simulink library "mpc555drivers"  (Simulink 6.0)
settings: Solver=ode45  SolverMode=SingleTasking  StartTime=0.0  StopTime=10.0  RelTol=1e-3
PreLoadFcn:
  | RTWConfigurationCB('preloadfcn', bdroot);
InitFcn:
  | % START RTW CONFIGURATION CODE %
  | RTWConfigurationCB('rtw_target_initfcn',gcs);
  | % END RTW CONFIGURATION CODE %
undefined symbols (not defined in the file or in its folder): pmax, scale
libraries: passthrough x52, driver_interface_library x18, mpc555toucan x11, mpc555extras x9, config_library x7, exprofilelib x4, simulink x3, mpc555drivers x2, canblocks x1
(part 1 of 3)
settings Model: Creator=The MathWorks Inc.  LastModifiedBy=batserve  ExtModeAutoUpdateStatusClock=off  ProdHWDeviceType=Specified
settings DataIOCC: SignalLoggingName=logsOut
settings OptimizationCC: BooleanDataType=off
settings DebuggingCC: CheckExecutionContextPreStartOutputMsg=on  CheckExecutionContextRuntimeOutputMsg=on  SolverPrmCheckMsg=none
settings HardwareCC: ProdHWDeviceType=Specified  TargetUnknown=on
settings ModelReferenceCC: UpdateModelReferenceTargets=IfOutOfDate

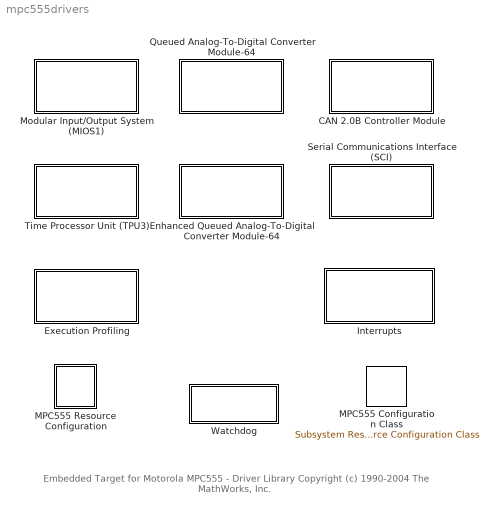
== system mpc555drivers ==
  note: Embedded Target for Motorola MPC555 - Driver Library
      | Copyright (c) 1990-2004 The MathWorks, Inc.
  CAN 2.0B Controller Module : Subsystem  PropExecContextAcrossSSBoundary=on
      mask Display: disp('TouCAN')
  Enhanced Queued Analog-To-Digital Converter Module-64 : Subsystem  PropExecContextAcrossSSBoundary=on
      mask Display: disp('QADC64E\n(MPC565/566)')
  Execution Profiling : Subsystem  PropExecContextAcrossSSBoundary=on
      mask Display: disp('Execution\nProfiling')
  Interrupts : Subsystem  PropExecContextAcrossSSBoundary=on
      settings: OpenFcn=mpc555interrupts
      mask Display: disp('Interrupt Handling')
  MPC555 Configuration Class : config_library/Subsystem Resource Configuration Class  Tag=CONFIGURATION DATA CLASS  dClassName=MPC555dkConfig.SYSTEM_CLOCKS  rClassName=MPC555dkConfig.SystemResources
  MPC555 Resource Configuration : Subsystem  Tag=RTW CONFIGURATION BLOCK  AncestorBlock=|  PropExecContextAcrossSSBoundary=on  mask(Subsystem Resource Configuration){oldParentName=, oldBlockName=, defaultConfigLibrary=}
      | config_library/Subsystem
      | Resource
      | Configuration
      mask prompts: oldParentName "Old Parent Name"; oldBlockName "Old Block Name"; defaultConfigLibrary "Default Configuration Library"
      settings: CopyFcn=RTWConfigurationCB('copyfcn',gcb);  DeleteFcn=RTWConfigurationCB('deletefcn',gcb);  UndoDeleteFcn=RTWConfigurationCB('NameChangeFcn',gcb);  PreSaveFcn=RTWConfigurationCB('presavefcn',gcb);  NameChangeFcn=RTWConfigurationCB('NameChangeFcn',gcb);  OpenFcn=RTWConfigurationCB('openfcn',gcb);
      mask Display: image(imread('target_icon.jpg'))
  Modular Input/Output System (MIOS1) : Subsystem  PropExecContextAcrossSSBoundary=on
      mask Display: disp(sprintf('MIOS1 / MIOS14'))
  Queued Analog-To-Digital Converter Module-64 : Subsystem  PropExecContextAcrossSSBoundary=on
      mask Display: disp('QADC64\n(MPC555)')
  Serial Communications Interface (SCI) : Subsystem  PropExecContextAcrossSSBoundary=on
      mask Display: disp('Serial')
  Time Processor Unit (TPU3) : Subsystem  PropExecContextAcrossSSBoundary=on
      mask Display: disp('TPU3')
  Watchdog : Subsystem  PropExecContextAcrossSSBoundary=on  mask(MPC555 Watchdog){timeout=0.1}
      mask prompts: timeout "Watchdog Timeout [seconds]"
      mask help:
      | Set the timeout period of the watchdog timer.
      |
      | Normally the timer is reset every time the fastest sample period of the model executes. If the model gets locked and stops executing then the watchdog will timeout and reset the processor.
      mask init:
      | [model_init_function_code] = mask_mpc555_watchdog('initfcn',gcb,timeout);
      mask Help: helpview([docroot '/toolbox/mpc555dk/mpc555dk.map'], 'Bow_Wow');
      mask CallbackString:
      | timeout = eval(get_param(gcb,'timeout'),[]);
      | % If eval returns empty, then it may be that a variable was
      | % specified rather than a numeric value. We can only do the range
      | % check at this point if a numeric value was entered.
      | if ~isempty(timeout)
      | 	timeout = mask_mpc555_watchdog('rangecheck',gcb,timeout);
      | end
      mask Display: disp('Watchdog \nTimer')

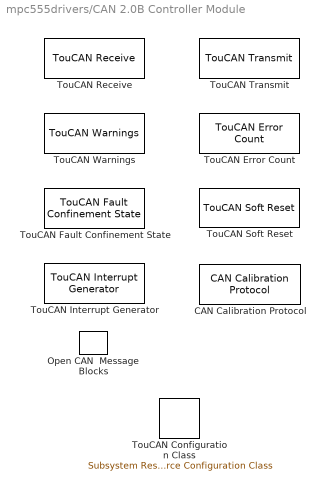
== system mpc555drivers/CAN 2.0B Controller Module ==
  CAN Calibration Protocol : mpc555toucan/CAN Calibration Protocol  CCP_STATION_ID=hex2dec('1')  module=A  ccp_cro_id=hex2dec('6FA')  ccp_cro_message_type=Extended (29-bit identifier)  ccp_return_id=hex2dec('6FB')  ccp_return_message_type=Extended (29-bit identifier)  TOTAL_NUM_ODTS=8  cro_sample_time=0.01
  Open CAN  Message Blocks : mpc555toucan/Open CAN  Message Blocks
  TouCAN Configuration Class : config_library/Subsystem Resource Configuration Class  Tag=CONFIGURATION DATA CLASS  dClassName=MPC555dkConfig.TOUCAN  rClassName=MPC555dkConfig.TOUCAN_RESOURCES
  TouCAN Error Count : mpc555toucan/TouCAN Error Count  module=A  t=0.1  enablePassThru=off
  TouCAN Fault Confinement State : mpc555toucan/TouCAN Fault Confinement State  module=A  t=0.1  enablePassThru=off
  TouCAN Interrupt Generator : mpc555toucan/TouCAN Interrupt Generator  module=A  callback=Error  float_flag=on
  TouCAN Receive : mpc555toucan/TouCAN Receive  module=A  ids=hex2dec('0001')  notification_type=Function Call Outport  auto_select_buffer=on  bufferids=14  use_queue=off  queue_length=3  message_type=Standard (11-bit identifier)  t=0.1
  TouCAN Soft Reset : mpc555toucan/TouCAN Soft Reset  module=A  t=-1
  TouCAN Transmit : mpc555toucan/TouCAN Transmit  module=A  tx_mode=Queued transmission with shared buffer  fifo_queue_length=8  bufferids=0  t=-1  enablePassThru=off
  TouCAN Warnings : mpc555toucan/TouCAN Warnings  module=A  t=0.1  enablePassThru=off

== system mpc555drivers/Enhanced Queued Analog-To-Digital Converter Module-64 ==
  QADCE Configuration Class : config_library/Subsystem Resource Configuration Class  Tag=CONFIGURATION DATA CLASS  dClassName=MPC555dkConfig.QADC64E  rClassName=MPC555dkConfig.QADC_Resources
  QADCE Analog In : Subsystem  PropExecContextAcrossSSBoundary=on  mask(MPC555 Analog Input (Enhanced QADC64, Continuous-scan)){module=A, channels=[ 44 45 46 47 64 65 66 ], justification=Right-justified (unsigned), t=0.1}
      mask prompts: module "QADCE module:"; t "Sample time:"
      mask help:
      | Analog input using one of the Queued Analog Digital Converter (QADC64) modules. The module is operated in continuous-scan mode.
      |
      | Specifying channel numbers:
      | - In non-multiplexed mode, specify the channels as a vector of numbers from [44..59, 64..87], correponding to pins AN44..AN59 and AN64..AN87.
      | - In multiplexed mode see the table in the documentation.
      mask init:
      | % check for a Resource Config block, and make sure it is MPC555
      | target = RTWConfigurationCB('get_target', gcb);
      | target.checkName('MPC555');
      | 
      | num_channels = length(channels);
      | register = mask_qadce_analogue_in(module,channels,justification);
      | 
      | if justification == 3
      |     outDType = 'int16';
      | else
      |    outDType = 'uint16';
      | end
      | 
      | % check for a valid target block
      | driverBlock = regexprep(gcb, sprintf('\n'), ' ');
      | target = RTWConfigurationCB('get_target', driverBlock);
      | 
      | % Perform Resource Configuration
      | RTWConfiguration.Target.acquireResourceForBlock(      ...
      |    gcb,                    ...   % Current block
      |    'MPC555dkConfig.QADC64E', ...   % Configuration Class
      |    'QADC_MODULES',          ...   % Resource Type associated with the configuration class
      |    module,                    ...   % Resource being requested
      |    'QADC Module'            ...   % Lable to be used in error messages
      | );
      mask Help: helpview([docroot '/toolbox/mpc555dk/mpc555dk.map'], 'QADCE_An_In');
      mask StyleString: popup(A|B),edit,popup(Right-justified (unsigned)|Left-justified (unsigned)|Left-justified (signed)),edit
      mask Display: disp(sprintf('Analog In\n(QADCE_%s)',module));
  QADCE Digital In : Subsystem  PropExecContextAcrossSSBoundary=on  mask(MPC555 Digital Input (Enhanced QADC64)){module=A, port=A, bits=[0 1 2 3], t=0.1}
      mask prompts: module "QADC module:"; t "Sample time:"
      mask help:
      | Digital input using one of the Queued Analog Digital Converter (QADC64) modules.
      |
      | Specify the bits you want to read as a vector of numbers from [0..7]. Depending on the selected port, the bits entered correspond to pins:
      | - PQA0..PQA7 (Port A)
      | - PQB0..PQB7 (Port B)
      mask init:
      | % check for a Resource Config block, and make sure it is MPC555
      | target = RTWConfigurationCB('get_target', gcb);
      | target.checkName('MPC555');
      | 
      | % check for a valid target block
      | driverBlock = regexprep(gcb, sprintf('\n'), ' ');
      | target = RTWConfigurationCB('get_target', driverBlock);
      | 
      | %parameter check
      | permitted = 0:7;
      | if any( ~ismember(bits,permitted) )
      |   error(['At least one illegal bit number number was specified. The permitted bit numbers are '...
      |          num2str(permitted) '. Check that all specified bit numbers are in this set.']);
      | end
      | 
      | % The Digital In Register To Read
      | register=['QADC_' module '.PORTQ' port '.R'];
      | 
      | % The Masks
      | masks = bitshift(1,bits,8);
      | 
      | % Perform Resource Configuration
      | for i = 1:length(bits)
      | 	pins{i} = sprintf('%d', bits(i));
      | end
      | resource = ['QADC_' module '_DIGITAL_PORT' port ];
      | RTWConfiguration.Target.acquireResourceForBlock(      ...
      |    gcb,                    ...   % Current block
      |    'MPC555dkConfig.QADC64E', ...   % Configuration Class
      |    resource,          ...   % Resource Type associated with the configuration class
      |    pins,                    ...   % Resources being requested
      |    'QADC Digital Input Pin(s)'            ...   % Lable to be used in error messages
      | );
      mask Help: helpview([docroot '/toolbox/mpc555dk/mpc555dk.map'], 'QADCE_Dig_In');
      mask StyleString: popup(A|B),popup(A|B),edit,edit
      mask Display: disp(sprintf('Digital In\n(QADCE_%s)',module));

== system mpc555drivers/Execution Profiling ==
  MPC555 Execution Profiling via CAN A : Subsystem  TreatAsAtomicUnit=on  PropExecContextAcrossSSBoundary=on  mask(MPC555 Execution Profiling via CAN Channel A){commandId=hex2dec('1FFFFF00'), execCopyFcn=on, dataId=hex2dec('1FFFFF01'), t=1}
      mask prompts: commandId "Start command CAN message identifier:"; execCopyFcn "Execute CopyFcn"; dataId "Returned data CAN message identifier:"; t "Sample time:"
      mask help:
      | Provides a CAN interface to the execution profiling engine. On receipt of a start command message, logging of execution profile data begins. On completion of a logging run, the recorded data is automatically returned via CAN.
      |
      | You must specify the message identifiers for the start command and the returned data. These identifiers must be compatible with the values used by the host-side part of the execution profiling utility. See also the MATLAB command profile_mpc555.
      mask init:
      | % check for a Resource Config block, and make sure it is MPC555
      | target = RTWConfigurationCB('get_target', gcb);
      | target.checkName('MPC555');
      settings: CopyFcn=exprofile_copyfcn(gcb);
      mask Help: helpview([docroot '/toolbox/mpc555dk/mpc555dk.map'], 'Execution_Profiling_Can_A');
      mask Display: disp('Execution Profiling\nvia CAN')
  MPC555 Execution Profiling via SCI1 : Subsystem  TreatAsAtomicUnit=on  PropExecContextAcrossSSBoundary=on  mask(MPC555  Execution Profiling via Serial Port SCI1){t=1, execCopyFcn=on}
      mask prompts: t "Sample time:"; execCopyFcn "Execute CopyFcn"
      mask help:
      | Provides a serial interface to the execution profiling engine. On receipt of a start command to the serial port, logging of execution profile data begins. On completion of a logging run, the recorded data is automatically returned via serial.
      |
      | No other serial blocks may be used in the model if an MPC555 Execution Profiling via SCI1 block is present.
      |
      | See also the MATLAB command profile_mpc555.
      mask init:
      | % check for a Resource Config block, and make sure it is MPC555
      | target = RTWConfigurationCB('get_target', gcb);
      | target.checkName('MPC555');
      settings: CopyFcn=exprofile_copyfcn(gcb);
      mask Help: helpview([docroot '/toolbox/mpc555/mpc555.map'], 'Execution_Profiling_SCI1');
      mask Display: disp('Execution Profiling\nvia Serial')

== system mpc555drivers/Interrupts ==

== system mpc555drivers/MPC555 Resource Configuration ==
  config : S-Function  FunctionName=sfunRTWConfig

== system mpc555drivers/Modular Input/Output System (MIOS1) ==
  MIOS Configuration Class : config_library/Subsystem Resource Configuration Class  Tag=CONFIGURATION DATA CLASS  dClassName=MPC555dkConfig.MIOS1  rClassName=MPC555dkConfig.MiosResources
  MIOS Digital In : Subsystem  PropExecContextAcrossSSBoundary=on  mask(MPC555 Digital Input (MPIOSM)){bits=[0 1 2], t=0.1, enablePassThru=off}
      mask prompts: t "Sample time:"; enablePassThru "Enable pass through (show simulation input)"
      mask help:
      | Reads the logical state of specified pins on the MIOS 16-bit parallel port I/O submodule (MPIOSM).
      |
      | Specify the bits you want to read as a vector of numbers from [0..15], corresponding to pins MPIO32B0..MPIO32B15.
      mask init:
      | simulinkPortControl(gcbh,'enable','PassThrough',enablePassThru);
      | 
      | %Deprecation warning for passthrough
      | if (enablePassThru)
      | 	passThroughDeprecationWarning;
      | end;
      | 
      | % check for a Resource Config block, and make sure it is MPC555
      | target = RTWConfigurationCB('get_target', gcb);
      | target.checkName('MPC555');
      | 
      | mpc555_mask_mios_dig_io('init', gcb, bits);
      | masks=uint16(bitshift(1,bits));
      | bits=int16(bits); % Prevent decimal points in generated code.
      mask Help: helpview([docroot '/toolbox/mpc555dk/mpc555dk.map'], 'MIOS_Dig_In');
      mask CallbackString: mpc555_mask_mios_dig_io('callback', gcb);||
      mask Display: disp(['Digital In\n(MPIOSM)'])
  MIOS Digital Out : Subsystem  PropExecContextAcrossSSBoundary=on  mask(MPC555 Digital Output (MPIOSM)){bits=[0 1], init=0, t=-1, enablePassThru=off}
      mask prompts: init "Initial output level:"; t "Sample time:"; enablePassThru "Enable pass through (show simulation output)"
      mask help:
      | Sets the logical state of specified pins on the MIOS 16-bit parallel port I/O submodule (MPIOSM). When the input signal is greater than zero a logical one is written to the corresponding pin; otherwise a logical zero is written.
      |
      | Specify the bits you want to set as a vector of numbers from [0..15], corresponding to pins MPIO32B0..MPIO32B15.
      mask init:
      | simulinkPortControl(gcbh,'enable','PassThrough',enablePassThru);
      | 
      | %Deprecation warning for passthrough
      | if (enablePassThru)
      | 	passThroughDeprecationWarning;
      | end;
      | 
      | bits = double(bits);
      | init = double(init~=0);
      | 
      | % Check the init and bits parameters for the correct length
      | if length(init) == 1
      | 	init = repmat(init,1,length(bits));
      | elseif length(init) ~= length(bits)
      | 	error('''Initial Output Level'' parameter must either be a scalar or the same length as the ''bits'' parameter.');
      | end
      | 
      | % check for a Resource Config block, and make sure it is MPC555
      | target = RTWConfigurationCB('get_target', gcb);
      | target.checkName('MPC555');
      | 
      | mpc555_mask_mios_dig_io('init', gcb, bits);
      | masks=uint16(bitshift(1,bits));
      mask Help: helpview([docroot '/toolbox/mpc555dk/mpc555dk.map'], 'MIOS_Dig_Out');
      mask CallbackString: mpc555_mask_mios_dig_io('callback', gcb);|||
      mask Display: disp(['Digital Out\n (MPIOSM)'])
  MIOS Digital Out (MPWMSM) : Subsystem  Priority=2  PropExecContextAcrossSSBoundary=on  mask(MPC555 Digital Output (MPWMSM)){module=0, init=0, t=-1, enablePassThru=off}
      mask prompts: module "MPWM submodule number:"; init "Initial output level:"; t "Sample time:"; enablePassThru "Enable pass through (show simulation output)"
      mask help:
      | Configures a MIOS pulse width modulation submodule (MPWMSM) for use as digital output. When the input signal is greater than zero a logical one is written to the output pin; otherwise a logical zero is written.
      |
      | This block outputs on one of the pins MPWM0..MPWM3 or MPWM16..MPWM19.
      mask init:
      | simulinkPortControl(gcbh,'enable','PassThrough',enablePassThru);
      | 
      | %Deprecation warning for passthrough
      | if (enablePassThru)
      | 	passThroughDeprecationWarning;
      | end;
      | 
      | % check for a Resource Config block, and make sure it is MPC555
      | target = RTWConfigurationCB('get_target', gcb);
      | target.checkName('MPC555');
      | 
      | init = init ~= 0;
      | 
      | % MIOS14 has 4 more PWM channels than the MIOS1
      | if ismember(module, {'4' '5' '20' '21'} ) && ...
      |    ~mpc555_module_available(mpc5xx_get_target_variant(gcb),'MIOS14')
      | 	msg = sprintf('\n\nPWM module %s is not available.\nModules { 4 5 20 21 } are only supported on processor variants with a MIOS14 module.\nPlease choose a different module or a different processor variant',module);
      | 	error(msg);
      | end
      | 
      | % Perform Resource Configuration
      | RTWConfiguration.Target.acquireResourceForBlock(      ...
      |    gcb,                    ...   % Current block
      |    'MPC555dkConfig.MIOS1', ...   % Configuration Class
      |    'PWM_MODULES',          ...   % Resource Type associated with the configuration class
      |    module,                    ...   % Resource being requested
      |    'PWM Module'            ...   % Label to be used in error messages
      | );
      mask Help: helpview([docroot '/toolbox/mpc555dk/mpc555dk.map'], 'MIOS_Dig_Out_MPWMSM');
      mask StyleString: popup(0|1|2|3|4|5|16|17|18|19|20|21),popup(0|1),edit,checkbox
      mask Display: disp('Digital Out\n(MPWMSM)')
  MIOS Pulse Width Modulation Out : Subsystem  Priority=2  PropExecContextAcrossSSBoundary=on  mask(MPC555 Pulse Width Modulation Output (MPWMSM)){module=0, timing_settings=off, period=0.0375, initpw=0.5, cp=, pp=, t=-1, pol=off, trsp=off, fren=off, enablePassThru=off}
      mask prompts: module "MPWM submodule number:"; timing_settings "Edit period registers manually"; period "Ideal period (sec):"; initpw "Initial duty cycle (0 <= duty cycle <= 1):"; cp "Clock prescaler field of MPWMSM Status/Control Register:"; pp "Number of clock ticks per period:"; t "Sample time:"; pol "Invert output polarity"; trsp "Activate transparent mode"; fren "Hold output when at debug breakpoint (freeze enable)"; enablePassThru "Enable pass through (show simulation output)"
      mask help:
      | Configures a MIOS pulse width modulation submodule (MPWMSM) to generate a pulse width modulated output signal.
      |
      | This block outputs on one of the pins MPWM0..MPWM3 or MPWM16..MPWM19.
      mask init:
      | simulinkPortControl(gcbh,'enable','PassThrough',enablePassThru);
      | 
      | %Deprecation warning for passthrough
      | if (enablePassThru)
      | 	passThroughDeprecationWarning;
      | end;
      | 
      | % check for a Resource Config block, and make sure it is MPC555
      | target = RTWConfigurationCB('get_target', gcb);
      | target.checkName('MPC555');
      | 
      | % Calculate period
      | [period,cp,pp] = mask_pwm_config('period_calc',gcb,period,cp,pp);
      | 
      | % Verify Initial pulse width
      | if initpw > 1 || initpw < 0
      | 	error('Initial Pulse Width Parameter ( pw ) must satisfy 0 <= pw <= 1');
      | end
      | % Calculate the initial value for the PULR register
      | initpw = round(pp * initpw);
      | 
      | % MIOS14 has 4 more PWM channels than the MIOS1
      | if ismember(module, {'4' '5' '20' '21'} ) && ...
      |    ~mpc555_module_available(mpc5xx_get_target_variant(gcb),'MIOS14')
      | 	msg = sprintf('\n\nPWM module %s is not available.\nModules { 4 5 20 21 } are only supported on processor variants with a MIOS14 module.\nPlease choose a different module or a different processor variant',module);
      | 	error(msg);
      | end
      | 
      | % Perform Resource Configuration
      | RTWConfiguration.Target.acquireResourceForBlock(      ...
      |    gcb,                    ...   % Current block
      |    'MPC555dkConfig.MIOS1', ...   % Configuration Class
      |    'PWM_MODULES',          ...   % Resource Type associated with the configuration class
      |    module,                    ...   % Resource being requested
      |    'PWM Module'            ...   % Lable to be used in error messages
      | );
      mask Help: helpview([docroot '/toolbox/mpc555dk/mpc555dk.map'], 'MIOS_PWM');
      mask StyleString: popup(0|1|2|3|4|5|16|17|18|19|20|21),checkbox,edit,edit,edit,edit,edit,checkbox,checkbox,checkbox,checkbox
      mask CallbackString: |mask_pwm_config('timing_settings',gcb)|mask_pwm_config('period_update',gcb)||mask_pwm_config('period_update',gcb)|mask_pwm_config('period_update',gcb)|||||
      mask Display: disp('PWM Out\n(MPWMSM)')
  MIOS Waveform Measurement : Subsystem  PropExecContextAcrossSSBoundary=on  mask(MPC555 Waveform Measurement (MDASM)){module=11, operation=Pulse width, bsl=Counter Bus 6 (CB6), range=[ 1e-006 , 0.065536 ], t=0.1, edpol=off, fren=off, enablePassThru=off}
      mask prompts: module "MDASM submodule number:"; operation "Measurement:"; bsl "Counter bus:"; range "Measurement range: [ resolution, max] seconds"; t "Sample time:"; edpol "Invert input polarity"; fren "Hold internal counters when at debug breakpoint (freeze enable)"; enablePassThru "Enable pass through (show simulation input)"
      mask help:
      | Configures the MIOS double action submodule (MDASM) for pulse width or pulse period measurement.
      |
      | This block inputs on one of the pins MDA11..MDA15 or MDA27..MDA31.
      mask init:
      | simulinkPortControl(gcbh,'enable','PassThrough',enablePassThru);
      | 
      | %Deprecation warning for passthrough
      | if (enablePassThru)
      | 	passThroughDeprecationWarning;
      | end;
      | 
      | % check for a Resource Config block, and make sure it is MPC555
      | target = RTWConfigurationCB('get_target', gcb);
      | target.checkName('MPC555');
      | 
      | % scale and pmax are
      | % all used under the mask
      | [scale, pmax, pmin] = mask_mdasm_ipwm('code',gcb);
      | 
      | % Perform Resource Configuration
      | RTWConfiguration.Target.acquireResourceForBlock(      ...
      |    gcb,                    ...   % Current block
      |    'MPC555dkConfig.MIOS1', ...   % Configuration Class
      |    'MDASM_MODULES',          ...   % Resource Type associated with the configuration class
      |    module,                    ...   % Resource being requested
      |    'MDASM Module'            ...   % Lable to be used in error messages
      | );
      mask Help: helpview([docroot '/toolbox/mpc555dk/mpc555dk.map'], 'Waveform_Measurement');
      mask StyleString: popup(11|12|13|14|15|27|28|29|30|31),popup(Pulse width|Pulse period),popup(Counter Bus 6 (CB6)|Counter Bus 22 (CB22)),edit,edit,checkbox,checkbox,checkbox
      mask CallbackString: ||mask_mdasm_ipwm('update_range', gcb);|||||
      mask Display: disp('Pulse Width\n(MDASM)');

== system mpc555drivers/Queued Analog-To-Digital Converter Module-64 ==
  QADC Configuration Class : config_library/Subsystem Resource Configuration Class  Tag=CONFIGURATION DATA CLASS  dClassName=MPC555dkConfig.QADC64  rClassName=MPC555dkConfig.QADC_Resources
  QADC Analog In : Subsystem  PropExecContextAcrossSSBoundary=on  mask(MPC555 Analog Input (QADC64, Continuous-scan)){module=A, channels=[0 1 2 3 48 49 50 51], justification=Right-justified (unsigned), t=0.1, enablePassThru=off}
      mask prompts: module "QADC module:"; t "Sample time:"; enablePassThru "Enable pass through (show simulation input)"
      mask help:
      | Analog input using one of the Queued Analog Digital Converter (QADC64) modules. The module is operated in continuous-scan mode.
      |
      | Specifying channel numbers:
      | - In non-multiplexed mode, specify the channels as a vector of numbers from [0..3, 48..59], correponding to pins AN0..AN3 and AN48..AN59.
      | - In multiplexed mode see the table in the documentation.
      mask init:
      | simulinkPortControl(gcbh,'enable','PassThrough',enablePassThru);
      | 
      | %Deprecation warning for passthrough
      | if (enablePassThru)
      | 	passThroughDeprecationWarning;
      | end;
      | 
      | % check for a Resource Config block, and make sure it is MPC555
      | target = RTWConfigurationCB('get_target', gcb);
      | target.checkName('MPC555');
      | 
      | num_channels = length(channels);
      | register = mask_qadc_analogue_in(module,channels,justification);
      | 
      | if justification == 3
      |     outDType = 'int16';
      | else
      |    outDType = 'uint16';
      | end
      | 
      | % check for a valid target block
      | driverBlock = regexprep(gcb, sprintf('\n'), ' ');
      | target = RTWConfigurationCB('get_target', driverBlock);
      | 
      | % Perform Resource Configuration
      | RTWConfiguration.Target.acquireResourceForBlock(      ...
      |    gcb,                    ...   % Current block
      |    'MPC555dkConfig.QADC64', ...   % Configuration Class
      |    'QADC_MODULES',          ...   % Resource Type associated with the configuration class
      |    module,                    ...   % Resource being requested
      |    'QADC Module'            ...   % Lable to be used in error messages
      | );
      mask Help: helpview([docroot '/toolbox/mpc555dk/mpc555dk.map'], 'QADC_An_In');
      mask StyleString: popup(A|B),edit,popup(Right-justified (unsigned)|Left-justified (unsigned)|Left-justified (signed)),edit,checkbox
      mask Display: disp(sprintf('Analog In\n(QADC_%s)',module));
  QADC Digital In : Subsystem  PropExecContextAcrossSSBoundary=on  mask(MPC555 Digital Input (QADC64)){module=A, port=A, bits=[0 1 2 3], t=0.1, enablePassThru=off}
      mask prompts: module "QADC module:"; t "Sample time:"; enablePassThru "Enable pass through (show simulation input)"
      mask help:
      | Digital input using one of the Queued Analog Digital Converter (QADC64) modules.
      |
      | Specify the bits you want to read as a vector of numbers from [0..7]. Depending on the selected port, the bits entered correspond to pins:
      | - PQA0..PQA7 (Port A)
      | - PQB0..PQB7 (Port B)
      mask init:
      | simulinkPortControl(gcbh,'enable','PassThrough',enablePassThru);
      | 
      | %Deprecation warning for passthrough
      | if (enablePassThru)
      | 	passThroughDeprecationWarning;
      | end;
      | 
      | % check for a Resource Config block, and make sure it is MPC555
      | target = RTWConfigurationCB('get_target', gcb);
      | target.checkName('MPC555');
      | 
      | % check for a valid target block
      | driverBlock = regexprep(gcb, sprintf('\n'), ' ');
      | target = RTWConfigurationCB('get_target', driverBlock);
      | 
      | %parameter check
      | permitted = 0:7;
      | if any( ~ismember(bits,permitted) )
      |   error(['At least one illegal bit number number was specified. The permitted bit numbers are '...
      |          num2str(permitted) '. Check that all specified bit numbers are in this set.']);
      | end
      | 
      | % The Digital In Register To Read
      | register=['QADC_' module '.PORTQ' port '.R'];
      | 
      | % The Masks
      | masks = bitshift(1,bits,8);
      | 
      | % Perform Resource Configuration
      | for i = 1:length(bits)
      | 	pins{i} = sprintf('%d', bits(i));
      | end
      | resource = ['QADC_' module '_DIGITAL_PORT' port ];
      | RTWConfiguration.Target.acquireResourceForBlock(      ...
      |    gcb,                    ...   % Current block
      |    'MPC555dkConfig.QADC64', ...   % Configuration Class
      |    resource,          ...   % Resource Type associated with the configuration class
      |    pins,                    ...   % Resources being requested
      |    'QADC Digital Input Pin(s)'            ...   % Lable to be used in error messages
      | );
      mask Help: helpview([docroot '/toolbox/mpc555dk/mpc555dk.map'], 'QADC_Dig_In');
      mask StyleString: popup(A|B),popup(A|B),edit,edit,checkbox
      mask Display: disp(sprintf('Digital In\n(QADC_%s)',module));

== system mpc555drivers/Serial Communications Interface (SCI) ==
  SCI Configuration Class : config_library/Subsystem Resource Configuration Class  Tag=CONFIGURATION DATA CLASS  dClassName=MPC555dkConfig.QSMCM  rClassName=""
  Serial Receive : S-Function  FunctionName=qsmcm_sci_rx  Parameters=T, module, show_length, max_length, show_reset, show_bytes_read, show_flags, show_overrun, buffer_size  mask(MPC555 Serial Communications Interface Receive){module=1, show_length=on, max_length=1, show_reset=off, show_bytes_read=on, show_flags=off, show_overrun=off, T=0.1}
      mask prompts: module "SCI module:"; show_length "Show input port for the requested number of bytes"; max_length "Maximum number of bytes:"; show_reset "Show reset port"; show_bytes_read "Show output port for the actual number of bytes read"; show_flags "Show framing error and parity error flags"; show_overrun "Show overrun flag"; T "Sample time:"
      mask help: Receive bytes over the Serial Communications Interface SCI1 or SCI2. Note that if the number of bytes available is smaller than the number of bytes requested then the actual number of bytes read is equal to the number of bytes available.
      mask init:
      | % check for a Resource Config block, and make sure it is MPC555
      | target = RTWConfigurationCB('get_target', gcb);
      | target.checkName('MPC555');
      | 
      | % Allocate the serial transmit interface
      | % Allocate the serial transmit interface
      | if module == 1
      |    buffer_size = 16;
      | else
      |    buffer_size = 1;
      | end
      | if round(max_length)~=max_length | max_length<1
      | 	error('The maximum length of data parameter must be a positive integer')
      | end
      | 
      | 
      | iconstr = mask_sci_rx(show_length, show_reset, show_bytes_read, show_flags, show_overrun);
      | set_param(gcb, 'MaskDisplay',iconstr);
      | 
      | % Perform Resource Configuration
      | sci_module = sprintf('SCI%d_RECEIVE',module);
      | RTWConfiguration.Target.acquireResourceForBlock(      ...
      |    gcb,                            ...   % Current block
      |    'MPC555dkConfig.SYSTEM_CLOCKS', ...   % Configuration Class
      |    'SERIAL_COMMUNICATIONS_INTERFACE',          ...   % Resource Type associated with the configuration class
      |    sci_module,                      ...   % Resource being requested
      |    'SCI Receive Module'            ...   % Lable to be used in error messages
      | );
      mask Help: helpview([docroot '/toolbox/mpc555dk/mpc555dk.map'], 'Serial_Receive');
      mask StyleString: popup(1|2),checkbox,edit,checkbox,checkbox,checkbox,checkbox,edit
      mask CallbackString:
      | |s = get_param(gcb,'show_length');
      | if strcmp(s,'on')
      |    simUtil_maskParam('show',gcb,'max_length');
      | else
      |    simUtil_maskParam('hide',gcb,'max_length');
      | end
      | ||||||
      mask Display: text(0.5, 0.5, ['SCI' num2str(module) '\nReceive'],'horizontalAlignment','center');port_label('output',1,'Data');port_label('input', 1, 'Len');port_label('output', 2, 'Num');
  Serial Transmit : S-Function  FunctionName=qsmcm_sci_tx  Parameters=T,show_length,show_num_sent, module, buffer_size  mask(SCI Transmit){module=1, show_length=on, show_num_sent=on, T=-1}
      mask prompts: module "SCI module:"; show_length "Show input port for the number of bytes to transmit"; show_num_sent "Show output port for the actual number of bytes transmitted"; T "Sample time:"
      mask help: Transmit bytes over the Serial Communications Interface SCI1 or SCI2. Note that if the number of available spaces in the buffer is smaller than the requested number of bytes to transmit then the actual number of bytes transmitted is equal to the number of spaces available.
      mask init:
      | % check for a Resource Config block, and make sure it is MPC555
      | target = RTWConfigurationCB('get_target', gcb);
      | target.checkName('MPC555');
      | 
      | % Allocate the serial transmit interface
      | if module == 1
      | 	buffer_size = 16;
      | else
      | 	buffer_size = 1;
      | end
      | 
      | iconstr = mask_sci_tx(show_length, show_num_sent);
      | set_param(gcb, 'MaskDisplay', iconstr);
      | 
      | 
      | % Perform Resource Configuration
      | sci_module = sprintf('SCI%d_TRANSMIT',module);
      | RTWConfiguration.Target.acquireResourceForBlock(      ...
      |    gcb,                            ...   % Current block
      |    'MPC555dkConfig.SYSTEM_CLOCKS', ...   % Configuration Class
      |    'SERIAL_COMMUNICATIONS_INTERFACE',          ...   % Resource Type associated with the configuration class
      |    sci_module,                      ...   % Resource being requested
      |    'SCI Transmit Module'            ...   % Lable to be used in error messages
      | );
      mask Help: helpview([docroot '/toolbox/mpc555dk/mpc555dk.map'], 'Serial_Transmit');
      mask StyleString: popup(1|2),checkbox,checkbox,edit
      mask Display: text(0.5, 0.5, ['SCI' num2str(module) '\nTransmit'],'horizontalAlignment','center'); port_label('input',1,'Data'); port_label('input', 2, 'Req');port_label('output', 1, 'Num');
